simulink model "IEEE30_case"  (R2024b)
settings: Solver=FixedStepAuto  StartTime=0  StopTime=5  FixedStep=1e-7  RelTol=1e-3
values from neighbouring files (symbols this model uses):
  GFL_DFIG_7_C_bus = 0.08    [IEEE30_case_parameters.m]
  GFL_DFIG_7_D_mutual = 2.500000e+3    (= 2500)    [IEEE30_case_parameters.m]
  GFL_DFIG_7_f0 = 60    [IEEE30_case_parameters.m]
  GFL_DFIG_7_gPLLi = 3200    [IEEE30_case_parameters.m]
  GFL_DFIG_7_gPLLp = 650    [IEEE30_case_parameters.m]
  GFL_DFIG_7_H_WT = 0.4    [IEEE30_case_parameters.m]
  GFL_DFIG_7_Hg = 0.8    [IEEE30_case_parameters.m]
  GFL_DFIG_7_Igq_ref = 0    [IEEE30_case_parameters.m]
  GFL_DFIG_7_Ird_ref = 704.45696    [IEEE30_case_parameters.m]
  GFL_DFIG_7_KI_V = -300000    [IEEE30_case_parameters.m]
  GFL_DFIG_7_KP_V = -1000    [IEEE30_case_parameters.m]
  GFL_DFIG_7_Ksh = 1.254300e+4    (= 12543)    [IEEE30_case_parameters.m]
  GFL_DFIG_7_Lg = 0.000483    [IEEE30_case_parameters.m]
  GFL_DFIG_7_Lm_pu = 4    [IEEE30_case_parameters.m]
  GFL_DFIG_7_N = 100    [IEEE30_case_parameters.m]
  GFL_DFIG_7_p = 2    [IEEE30_case_parameters.m]
  GFL_DFIG_7_Pitch = 0    [IEEE30_case_parameters.m]
  GFL_DFIG_7_R = 44    [IEEE30_case_parameters.m]
  GFL_DFIG_7_Rg = 2.000000e-5    (= 2e-05)    [IEEE30_case_parameters.m]
  GFL_DFIG_7_rho = 1.225    [IEEE30_case_parameters.m]
  GFL_DFIG_7_rPLLi = 4500    [IEEE30_case_parameters.m]
  GFL_DFIG_7_rPLLp = 620    [IEEE30_case_parameters.m]
  GFL_DFIG_7_Rs_pu = 0.011    [IEEE30_case_parameters.m]
  GFL_DFIG_7_Sbase = 2.000000e+6    (= 2000000)    [IEEE30_case_parameters.m]
  GFL_DFIG_7_ugq_ref = 0    [IEEE30_case_parameters.m]
  GFL_DFIG_7_usd_ref = 0    [IEEE30_case_parameters.m]
  GFL_DFIG_7_Vbase = 690    [IEEE30_case_parameters.m]
  GFL_DFIG_7_Vdc_ref = 1200    [IEEE30_case_parameters.m]
  GFL_DFIG_7_wind = 12    [IEEE30_case_parameters.m]
  GFL_DFIG_7_wm_ref = 518.184209    [IEEE30_case_parameters.m]
  SG_D_13_D = 0.01056    [IEEE30_case_parameters.m]
  SG_D_13_EnableSaturation = 0    [IEEE30_case_parameters.m]
  SG_D_13_f0 = 60    [IEEE30_case_parameters.m]
  SG_D_13_H = 7.5    [IEEE30_case_parameters.m]
  SG_D_13_K_A = 20    [IEEE30_case_parameters.m]
  SG_D_13_K_E = 1.000000e+1    (= 10)    [IEEE30_case_parameters.m]
  SG_D_13_K_F = 2.363    [IEEE30_case_parameters.m]
  SG_D_13_K_s = 0.5    [IEEE30_case_parameters.m]
  SG_D_13_R_a = 0.001088    [IEEE30_case_parameters.m]
  SG_D_13_S_A = 1    [IEEE30_case_parameters.m]
  SG_D_13_S_B = 0.103    [IEEE30_case_parameters.m]
  SG_D_13_S_N = 10.659857    [IEEE30_case_parameters.m]
  SG_D_13_SpeedPara = 200    [IEEE30_case_parameters.m]
  SG_D_13_T_0 = 0.370163    [IEEE30_case_parameters.m]
  SG_D_13_T_1 = 0.3    [IEEE30_case_parameters.m]
  SG_D_13_T_2 = 0.05    [IEEE30_case_parameters.m]
  SG_D_13_T_3 = 0.02    [IEEE30_case_parameters.m]
  SG_D_13_T_4 = 0.005    [IEEE30_case_parameters.m]
  SG_D_13_T_A = 0.02    [IEEE30_case_parameters.m]
  SG_D_13_T_dd = 8.000000e+0    (= 8)    [IEEE30_case_parameters.m]
  SG_D_13_T_ddd = 0.04    [IEEE30_case_parameters.m]
  SG_D_13_T_E = 0.314    [IEEE30_case_parameters.m]
  SG_D_13_T_F = 0.35    [IEEE30_case_parameters.m]
  SG_D_13_T_qd = 0.8    [IEEE30_case_parameters.m]
  SG_D_13_T_qdd = 0.02    [IEEE30_case_parameters.m]
  SG_D_13_T_speed = 0.1    [IEEE30_case_parameters.m]
  SG_D_13_T_w = 0.5    [IEEE30_case_parameters.m]
  SG_D_13_V_ref = 1.696619    [IEEE30_case_parameters.m]
  SG_D_13_w_ref = 376.991118    [IEEE30_case_parameters.m]
  SG_D_13_x_d = 1.9    [IEEE30_case_parameters.m]
  SG_D_13_x_dd = 0.302    [IEEE30_case_parameters.m]
  SG_D_13_x_ddd = 0.204    [IEEE30_case_parameters.m]
  SG_D_13_x_l = 0.05    [IEEE30_case_parameters.m]
  SG_D_13_x_q = 1.3    [IEEE30_case_parameters.m]
  SG_D_13_x_qd = 0.5    [IEEE30_case_parameters.m]
  SG_D_13_x_qdd = 0.3    [IEEE30_case_parameters.m]
  SG_D_1_D = 0.01056    [IEEE30_case_parameters.m]
  SG_D_1_EnableSaturation = 0    [IEEE30_case_parameters.m]
  SG_D_1_f0 = 60    [IEEE30_case_parameters.m]
  SG_D_1_H = 7.5    [IEEE30_case_parameters.m]
  SG_D_1_K_A = 20    [IEEE30_case_parameters.m]
  SG_D_1_K_E = 1.000000e+1    (= 10)    [IEEE30_case_parameters.m]
  SG_D_1_K_F = 2.363    [IEEE30_case_parameters.m]
  SG_D_1_K_s = 0.5    [IEEE30_case_parameters.m]
  SG_D_1_R_a = 0.001088    [IEEE30_case_parameters.m]
  SG_D_1_S_A = 1    [IEEE30_case_parameters.m]
  SG_D_1_S_B = 0.103    [IEEE30_case_parameters.m]
  SG_D_1_S_N = 10.659857    [IEEE30_case_parameters.m]
  SG_D_1_SpeedPara = 200    [IEEE30_case_parameters.m]
  SG_D_1_T_0 = 0.259812    [IEEE30_case_parameters.m]
  SG_D_1_T_1 = 0.3    [IEEE30_case_parameters.m]
  SG_D_1_T_2 = 0.05    [IEEE30_case_parameters.m]
  SG_D_1_T_3 = 0.02    [IEEE30_case_parameters.m]
  SG_D_1_T_4 = 0.005    [IEEE30_case_parameters.m]
  SG_D_1_T_A = 0.02    [IEEE30_case_parameters.m]
  SG_D_1_T_dd = 8.000000e+0    (= 8)    [IEEE30_case_parameters.m]
  SG_D_1_T_ddd = 0.04    [IEEE30_case_parameters.m]
  SG_D_1_T_E = 0.314    [IEEE30_case_parameters.m]
  SG_D_1_T_F = 0.35    [IEEE30_case_parameters.m]
  SG_D_1_T_qd = 0.8    [IEEE30_case_parameters.m]
  SG_D_1_T_qdd = 0.02    [IEEE30_case_parameters.m]
  SG_D_1_T_speed = 0.1    [IEEE30_case_parameters.m]
  SG_D_1_T_w = 0.5    [IEEE30_case_parameters.m]
  SG_D_1_V_ref = 1.544107    [IEEE30_case_parameters.m]
  SG_D_1_w_ref = 376.991118    [IEEE30_case_parameters.m]
  SG_D_1_x_d = 1.9    [IEEE30_case_parameters.m]
  SG_D_1_x_dd = 0.302    [IEEE30_case_parameters.m]
  SG_D_1_x_ddd = 0.204    [IEEE30_case_parameters.m]
  SG_D_1_x_l = 0.05    [IEEE30_case_parameters.m]
  SG_D_1_x_q = 1.3    [IEEE30_case_parameters.m]
  SG_D_1_x_qd = 0.5    [IEEE30_case_parameters.m]
  SG_D_1_x_qdd = 0.3    [IEEE30_case_parameters.m]
  SG_D_22_D = 0.01056    [IEEE30_case_parameters.m]
  SG_D_22_EnableSaturation = 0    [IEEE30_case_parameters.m]
  SG_D_22_f0 = 60    [IEEE30_case_parameters.m]
  SG_D_22_H = 7.5    [IEEE30_case_parameters.m]
  SG_D_22_K_A = 20    [IEEE30_case_parameters.m]
  SG_D_22_K_E = 1.000000e+1    (= 10)    [IEEE30_case_parameters.m]
  SG_D_22_K_F = 2.363    [IEEE30_case_parameters.m]
  SG_D_22_K_s = 0.5    [IEEE30_case_parameters.m]
  SG_D_22_R_a = 0.001088    [IEEE30_case_parameters.m]
  SG_D_22_S_A = 1    [IEEE30_case_parameters.m]
  SG_D_22_S_B = 0.103    [IEEE30_case_parameters.m]
  SG_D_22_S_N = 10.659857    [IEEE30_case_parameters.m]
  SG_D_22_SpeedPara = 200    [IEEE30_case_parameters.m]
  SG_D_22_T_0 = 0.216121    [IEEE30_case_parameters.m]
  SG_D_22_T_1 = 0.3    [IEEE30_case_parameters.m]
  SG_D_22_T_2 = 0.05    [IEEE30_case_parameters.m]
  SG_D_22_T_3 = 0.02    [IEEE30_case_parameters.m]
  SG_D_22_T_4 = 0.005    [IEEE30_case_parameters.m]
  ... (+126 more)
(part 22 of 27)

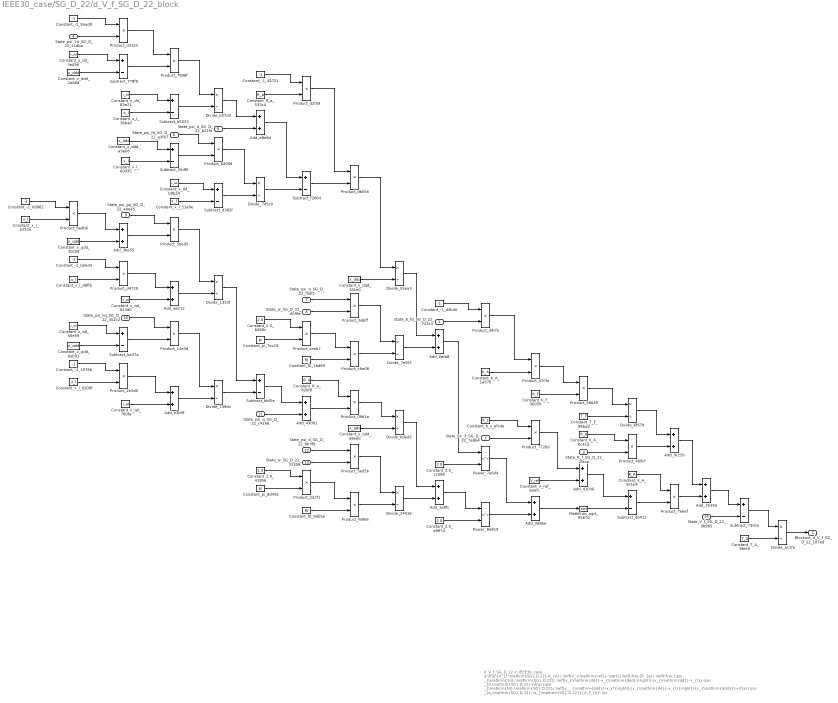
== system IEEE30_case/SG_D_22/d_V_f_SG_D_22_block ==
  note: d_V_f_SG_D_22 in IEEE30_case
      | $-\frac{V_{f,\mathrm{SG},D,22}-K_{A}\,\left(V_{\mathrm{ref}}-\sqrt{{\left(\frac{R_{a}\,\left(\frac{\psi _{\mathrm{1d},\mathrm{SG},D,22}\,\left(x_{\mathrm{dd}}-x_{\mathrm{ddd}}\right)}{x_{\mathrm{dd}}-x_{l}}-\psi _{d,\mathrm{SG},D,22}+\frac{\psi _{\mathrm{fd},\mathrm{SG},D,22}\,\left(x_{\mathrm{ddd}}-x_{l}\right)}{x_{\mathrm{dd}}-x_{l}}\right)}{x_{\mathrm{ddd}}}+\frac{\psi _{q,\mathrm{SG},D,22}\,w_{\mathrm{SG},D,22}}{2\,f_{0}\,\pi }\right)}^2+{\left(\frac{R_{a}\,\left(\psi _{q,\mathrm{SG},D,22}+\frac{\psi _{\mathrm{gq},\mathrm{SG},D,22}\,\left(x_{l}-x_{\mathrm{qdd}}\right)}{x_{l}-x_{\mathrm{qd}}}+\frac{\psi _{\mathrm{kq},\mathrm{SG},D,22}\,\left(x_{\mathrm{qd}}-x_{\mathrm{qdd}}\right)}{x_{l}-x_{\mathrm{qd}}}\right)}{x_{\mathrm{qdd}}}+\frac{\psi _{d,\mathrm{SG},D,22}\,w_{\mathrm{SG},D,22}}{2\,f_{0}\,\pi }\right)}^2}+K_{s}\,\mathrm{Px}_{3,\mathrm{SG},D,22}\right)-K_{A}\,R_{f,\mathrm{SG},D,22}+\frac{E_{\mathrm{fd},\mathrm{SG},D,22}\,K_{A}\,K_{F}}{T_{F}}}{T_{A}}$
      | Automatically generated on 2025-11-01 18:36:26 .
  State_E_fd_SG_D_22_743c3 : Inport
  State_R_f_SG_D_22_2faca : Inport  Port=2
  State_Px_3_SG_D_22_7a9b4 : Inport  Port=3
  State_psi_1d_SG_D_22_11dba : Inport  Port=4
  State_psi_d_SG_D_22_b21fa : Inport  Port=5
  State_psi_fd_SG_D_22_e3f07 : Inport  Port=6
  State_psi_q_SG_D_22_f5df1 : Inport  Port=7
  State_w_SG_D_22_d59fe : Inport  Port=8
  State_psi_gq_SG_D_22_abe45 : Inport  Port=9
  State_psi_kq_SG_D_22_352c2 : Inport  Port=10
  State_psi_q_SG_D_22_c4168 : Inport  Port=11
  State_psi_d_SG_D_22_8b3f8 : Inport  Port=12
  State_w_SG_D_22_31356 : Inport  Port=13
  State_V_f_SG_D_22_db965 : Inport  Port=14
  Add_0efa8 : Sum
  Add_1e8fc : Sum
  Add_3539d : Sum
  Add_3be55 : Sum
  Add_3d8ee : Sum
  Add_41036 : Sum
  Add_43081 : Sum
  Add_9cc50 : Sum
  Add_a6212 : Sum
  Add_e3b9f : Sum
  Add_e8e6d : Sum
  Constant_-1_0d962 : Constant  Value=-1
  Constant_-1_1978b : Constant  Value=-1
  Constant_-1_44751 : Constant  Value=-1
  Constant_-1_9aad8 : Constant  Value=-1
  Constant_-1_bb5d4 : Constant  Value=-1
  Constant_-1_d3b46 : Constant  Value=-1
  Constant_2.0_41856 : Constant  Value=2.0
  Constant_2.0_a9874 : Constant  Value=2.0
  Constant_2.0_b068c : Constant  Value=2.0
  Constant_2.0_cc098 : Constant  Value=2.0
  Constant_K_A_0c41a : Constant  Value=K_A
  Constant_K_A_1a676 : Constant  Value=K_A
  Constant_K_A_8c1b4 : Constant  Value=K_A
  Constant_K_F_36050 : Constant  Value=K_F
  Constant_K_s_afc4e : Constant  Value=K_s
  Constant_R_a_533c4 : Constant  Value=R_a
  Constant_R_a_82bf8 : Constant  Value=R_a
  Constant_T_A_9fe59 : Constant  Value=T_A
  Constant_T_F_98bad : Constant  Value=T_F
  Constant_V_ref_6e5fc : Constant  Value=V_ref
  Constant_f0_1bd69 : Constant  Value=f0
  Constant_f0_9db5e : Constant  Value=f0
  Constant_pi_7ac18 : Constant  Value=pi
  Constant_pi_8d43a : Constant  Value=pi
  Constant_x_dd_83e21 : Constant  Value=x_dd
  Constant_x_dd_b9b24 : Constant  Value=x_dd
  Constant_x_dd_fe496 : Constant  Value=x_dd
  Constant_x_ddd_191e0 : Constant  Value=x_ddd
  Constant_x_ddd_2a6b8 : Constant  Value=x_ddd
  Constant_x_ddd_a3e68 : Constant  Value=x_ddd
  Constant_x_l_38b4d : Constant  Value=x_l
  Constant_x_l_51a9e : Constant  Value=x_l
  Constant_x_l_60d35 : Constant  Value=x_l
  Constant_x_l_d208f : Constant  Value=x_l
  Constant_x_l_d6ffb : Constant  Value=x_l
  Constant_x_l_e152e : Constant  Value=x_l
  Constant_x_qd_56e59 : Constant  Value=x_qd
  Constant_x_qd_760fa : Constant  Value=x_qd
  Constant_x_qd_813d0 : Constant  Value=x_qd
  Constant_x_qdd_0eb91 : Constant  Value=x_qdd
  Constant_x_qdd_30cb9 : Constant  Value=x_qdd
  Constant_x_qdd_d8eeb : Constant  Value=x_qdd
  Divide_1353f : Product  Inputs=*/
  Divide_24016 : Product  Inputs=*/
  Divide_55ea3 : Product  Inputs=*/
  Divide_6f679 : Product  Inputs=*/
  Divide_749cb : Product  Inputs=*/
  Divide_7d5c0 : Product  Inputs=*/
  Divide_7e91f : Product  Inputs=*/
  Divide_ac1fa : Product  Inputs=*/
  Divide_b57d3 : Product  Inputs=*/
  Divide_bded9 : Product  Inputs=*/
  MathFunc_sqrt_95670 : Sqrt
  Power_7a6d4 : Math  Operator=pow
  Power_8e819 : Math  Operator=pow
  Product_0961a : Product
  Product_14e3d : Product
  Product_2d2f1 : Product
  Product_2e2d0 : Product
  Product_469cf : Product
  Product_47f3a : Product
  Product_56649 : Product
  Product_5ed5b : Product
  Product_5eed5 : Product
  Product_6409d : Product
  Product_7726d : Product
  Product_7848f : Product
  Product_7e6ef : Product
  Product_8adb6 : Product
  Product_9dbff : Product
  Product_c6e08 : Product
  Product_ceab7 : Product
  Product_d2f59 : Product
  Product_d31e3 : Product
  Product_d4729 : Product
  Product_d4cfa : Product
  Product_db056 : Product
  Product_f69e6 : Product
  Subtract_35df0 : Sum  Inputs=+-
  Subtract_730ce : Sum  Inputs=+-
  Subtract_778f9 : Sum  Inputs=+-
  Subtract_b5033 : Sum  Inputs=+-
  Subtract_ba37a : Sum  Inputs=+-
  Subtract_bbf2a : Sum  Inputs=+-
  Subtract_d0412 : Sum  Inputs=+-
  Subtract_d382f : Sum  Inputs=+-
  Subtract_f2864 : Sum  Inputs=+-
  Blockout_d_V_f_SG_D_22_187ed : Outport
  wires:
  Constant_-1_0d962/1 -> Product_8adb6/1
  Product_8adb6/1 -> Add_3be55/1
  Constant_x_l_e152e/1 -> Product_8adb6/2
  Product_d31e3/1 -> Product_7848f/1
  Constant_-1_9aad8/1 -> Product_d31e3/1
  Subtract_778f9/1 -> Product_7848f/2
  Constant_x_dd_fe496/1 -> Subtract_778f9/1
  Product_6409d/1 -> Divide_7d5c0/1
  State_psi_1d_SG_D_22_11dba/1 -> Product_d31e3/2
  Constant_x_qdd_30cb9/1 -> Add_3be55/2
  State_psi_q_SG_D_22_f5df1/1 -> Product_9dbff/1
  Constant_x_ddd_2a6b8/1 -> Subtract_778f9/2
  Product_d4729/1 -> Add_a6212/1
  Constant_-1_bb5d4/1 -> Product_d4729/1
  Product_ceab7/1 -> Product_c6e08/1
  Constant_x_l_d6ffb/1 -> Product_d4729/2
  Constant_2.0_b068c/1 -> Product_ceab7/1
  Subtract_ba37a/1 -> Product_14e3d/2
  Constant_x_qd_56e59/1 -> Subtract_ba37a/1
  Subtract_bbf2a/1 -> Add_43081/1
  Constant_x_qdd_0eb91/1 -> Subtract_ba37a/2
  Constant_-1_44751/1 -> Product_d2f59/1
  Product_2e2d0/1 -> Add_e3b9f/1
  Constant_-1_1978b/1 -> Product_2e2d0/1
  Constant_x_dd_b9b24/1 -> Subtract_d382f/1
  Constant_x_l_d208f/1 -> Product_2e2d0/2
  Constant_2.0_41856/1 -> Product_2d2f1/1
  Subtract_b5033/1 -> Divide_b57d3/2
  Constant_x_dd_83e21/1 -> Subtract_b5033/1
  Constant_pi_8d43a/1 -> Product_2d2f1/2
  Constant_x_l_38b4d/1 -> Subtract_b5033/2
  Constant_x_qd_760fa/1 -> Add_e3b9f/2
  Constant_x_ddd_a3e68/1 -> Subtract_35df0/1
  Subtract_f2864/1 -> Product_db056/2
  Constant_x_l_60d35/1 -> Subtract_35df0/2
  Product_5eed5/1 -> Divide_1353f/1
  State_psi_gq_SG_D_22_abe45/1 -> Product_5eed5/1
  Add_3be55/1 -> Product_5eed5/2
  Constant_x_qd_813d0/1 -> Add_a6212/2
  Product_14e3d/1 -> Divide_749cb/1
  State_psi_kq_SG_D_22_352c2/1 -> Product_14e3d/1
  Product_7848f/1 -> Divide_b57d3/1
  State_psi_fd_SG_D_22_e3f07/1 -> Product_6409d/1
  State_psi_q_SG_D_22_c4168/1 -> Add_43081/2
  Subtract_35df0/1 -> Product_6409d/2
  Constant_x_l_51a9e/1 -> Subtract_d382f/2
  Constant_f0_1bd69/1 -> Product_c6e08/2
  Add_a6212/1 -> Divide_1353f/2
  Product_d2f59/1 -> Product_db056/1
  Add_e3b9f/1 -> Divide_749cb/2
  Divide_b57d3/1 -> Add_e8e6d/1
  State_psi_d_SG_D_22_b21fa/1 -> Add_e8e6d/2
  Constant_R_a_533c4/1 -> Product_d2f59/2
  Subtract_d382f/1 -> Divide_7d5c0/2
  Divide_1353f/1 -> Subtract_bbf2a/1
  Divide_749cb/1 -> Subtract_bbf2a/2
  Add_e8e6d/1 -> Subtract_f2864/1
  Divide_7d5c0/1 -> Subtract_f2864/2
  Constant_pi_7ac18/1 -> Product_ceab7/2
  State_w_SG_D_22_d59fe/1 -> Product_9dbff/2
  Constant_R_a_82bf8/1 -> Product_0961a/1
  Add_43081/1 -> Product_0961a/2
  State_psi_d_SG_D_22_8b3f8/1 -> Product_5ed5b/1
  State_w_SG_D_22_31356/1 -> Product_5ed5b/2
  Product_2d2f1/1 -> Product_f69e6/1
  Constant_f0_9db5e/1 -> Product_f69e6/2
  Product_db056/1 -> Divide_55ea3/1
  Constant_x_ddd_191e0/1 -> Divide_55ea3/2
  Product_9dbff/1 -> Divide_7e91f/1
  Product_c6e08/1 -> Divide_7e91f/2
  Product_0961a/1 -> Divide_bded9/1
  Constant_x_qdd_d8eeb/1 -> Divide_bded9/2
  Product_5ed5b/1 -> Divide_24016/1
  Product_f69e6/1 -> Divide_24016/2
  Constant_K_A_1a676/1 -> Product_47f3a/2
  Divide_55ea3/1 -> Add_0efa8/1
  Divide_7e91f/1 -> Add_0efa8/2
  Divide_bded9/1 -> Add_1e8fc/1
  Divide_24016/1 -> Add_1e8fc/2
  Constant_-1_d3b46/1 -> Product_d4cfa/1
  State_E_fd_SG_D_22_743c3/1 -> Product_d4cfa/2
  Add_0efa8/1 -> Power_7a6d4/1
  Constant_2.0_cc098/1 -> Power_7a6d4/2
  Add_1e8fc/1 -> Power_8e819/1
  Constant_2.0_a9874/1 -> Power_8e819/2
  Product_d4cfa/1 -> Product_47f3a/1
  Constant_K_s_afc4e/1 -> Product_7726d/1
  State_Px_3_SG_D_22_7a9b4/1 -> Product_7726d/2
  Power_7a6d4/1 -> Add_3d8ee/1
  Power_8e819/1 -> Add_3d8ee/2
  Product_47f3a/1 -> Product_56649/1
  Add_3d8ee/1 -> MathFunc_sqrt_95670/1
  Constant_K_F_36050/1 -> Product_56649/2
  Product_7726d/1 -> Add_41036/1
  Constant_V_ref_6e5fc/1 -> Add_41036/2
  Product_56649/1 -> Divide_6f679/1
  Constant_T_F_98bad/1 -> Divide_6f679/2
  Constant_K_A_0c41a/1 -> Product_469cf/1
  State_R_f_SG_D_22_2faca/1 -> Product_469cf/2
  Add_41036/1 -> Subtract_d0412/1
  MathFunc_sqrt_95670/1 -> Subtract_d0412/2
  Divide_6f679/1 -> Add_9cc50/1
  Product_469cf/1 -> Add_9cc50/2
  Constant_K_A_8c1b4/1 -> Product_7e6ef/1
  Subtract_d0412/1 -> Product_7e6ef/2
  Add_9cc50/1 -> Add_3539d/1
  Product_7e6ef/1 -> Add_3539d/2
  Add_3539d/1 -> Subtract_730ce/1
  State_V_f_SG_D_22_db965/1 -> Subtract_730ce/2
  Subtract_730ce/1 -> Divide_ac1fa/1
  Constant_T_A_9fe59/1 -> Divide_ac1fa/2
  Divide_ac1fa/1 -> Blockout_d_V_f_SG_D_22_187ed/1

== system IEEE30_case/SG_D_22/d_psi_1d_SG_D_22_block ==
  note: d_psi_1d_SG_D_22 in IEEE30_case
      | $-\frac{\psi _{\mathrm{1d},\mathrm{SG},D,22}-\psi _{\mathrm{fd},\mathrm{SG},D,22}+\frac{\left(x_{\mathrm{dd}}-x_{l}\right)\,\left(\frac{\psi _{\mathrm{1d},\mathrm{SG},D,22}\,\left(x_{\mathrm{dd}}-x_{\mathrm{ddd}}\right)}{x_{\mathrm{dd}}-x_{l}}-\psi _{d,\mathrm{SG},D,22}+\frac{\psi _{\mathrm{fd},\mathrm{SG},D,22}\,\left(x_{\mathrm{ddd}}-x_{l}\right)}{x_{\mathrm{dd}}-x_{l}}\right)}{x_{\mathrm{ddd}}}}{T_{\mathrm{ddd}}}$
      | Automatically generated on 2025-11-01 18:36:01 .
  State_psi_1d_SG_D_22_172da : Inport
  State_psi_fd_SG_D_22_c2d5a : Inport  Port=2
  State_psi_1d_SG_D_22_e0ab6 : Inport  Port=3
  State_psi_d_SG_D_22_a4972 : Inport  Port=4
  State_psi_fd_SG_D_22_3322a : Inport  Port=5
  Add_5a731 : Sum
  Add_823bb : Sum
  Add_8bdee : Sum
  Constant_-1_43b70 : Constant  Value=-1
  Constant_-1_e3690 : Constant  Value=-1
  Constant_T_ddd_16786 : Constant  Value=T_ddd
  Constant_x_dd_2a533 : Constant  Value=x_dd
  Constant_x_dd_3a236 : Constant  Value=x_dd
  Constant_x_dd_89937 : Constant  Value=x_dd
  Constant_x_dd_d0c64 : Constant  Value=x_dd
  Constant_x_ddd_40c6f : Constant  Value=x_ddd
  Constant_x_ddd_7eefb : Constant  Value=x_ddd
  Constant_x_ddd_b7266 : Constant  Value=x_ddd
  Constant_x_l_19e50 : Constant  Value=x_l
  Constant_x_l_5eccd : Constant  Value=x_l
  Constant_x_l_88938 : Constant  Value=x_l
  Constant_x_l_d4803 : Constant  Value=x_l
  Divide_10e07 : Product  Inputs=*/
  Divide_5218a : Product  Inputs=*/
  Divide_a8712 : Product  Inputs=*/
  Divide_da239 : Product  Inputs=*/
  Product_011ec : Product
  Product_57d84 : Product
  Product_6887b : Product
  Product_99b88 : Product
  Product_9d3cd : Product
  Subtract_1db70 : Sum  Inputs=+-
  Subtract_59386 : Sum  Inputs=+-
  Subtract_5a27d : Sum  Inputs=+-
  Subtract_b5060 : Sum  Inputs=+-
  Subtract_b7795 : Sum  Inputs=+-
  Subtract_e43cc : Sum  Inputs=+-
  Blockout_d_psi_1d_SG_D_22_39dbc : Outport
  wires:
  Constant_-1_e3690/1 -> Product_9d3cd/1
  State_psi_1d_SG_D_22_e0ab6/1 -> Product_9d3cd/2
  Constant_x_l_88938/1 -> Subtract_59386/2
  Subtract_b5060/1 -> Product_6887b/2
  Constant_x_dd_2a533/1 -> Subtract_1db70/1
  Product_9d3cd/1 -> Product_99b88/1
  Divide_5218a/1 -> Subtract_5a27d/2
  Constant_x_ddd_40c6f/1 -> Subtract_1db70/2
  Subtract_1db70/1 -> Product_99b88/2
  State_psi_d_SG_D_22_a4972/1 -> Add_8bdee/2
  Subtract_b7795/1 -> Divide_da239/2
  Constant_x_dd_89937/1 -> Subtract_b7795/1
  Constant_x_l_d4803/1 -> Subtract_b7795/2
  Constant_x_ddd_b7266/1 -> Subtract_b5060/1
  Add_5a731/1 -> Divide_a8712/1
  Constant_x_l_5eccd/1 -> Subtract_b5060/2
  Product_99b88/1 -> Divide_da239/1
  State_psi_fd_SG_D_22_3322a/1 -> Product_6887b/1
  Constant_x_dd_3a236/1 -> Subtract_e43cc/1
  Constant_x_l_19e50/1 -> Subtract_e43cc/2
  Divide_da239/1 -> Add_8bdee/1
  Product_6887b/1 -> Divide_5218a/1
  Subtract_e43cc/1 -> Divide_5218a/2
  Constant_x_dd_d0c64/1 -> Subtract_59386/1
  Add_8bdee/1 -> Subtract_5a27d/1
  Constant_-1_43b70/1 -> Product_011ec/1
  Add_823bb/1 -> Add_5a731/1
  State_psi_1d_SG_D_22_172da/1 -> Product_011ec/2
  Subtract_59386/1 -> Product_57d84/1
  Divide_10e07/1 -> Add_5a731/2
  Subtract_5a27d/1 -> Product_57d84/2
  Product_011ec/1 -> Add_823bb/1
  State_psi_fd_SG_D_22_c2d5a/1 -> Add_823bb/2
  Product_57d84/1 -> Divide_10e07/1
  Constant_x_ddd_7eefb/1 -> Divide_10e07/2
  Divide_a8712/1 -> Blockout_d_psi_1d_SG_D_22_39dbc/1
  Constant_T_ddd_16786/1 -> Divide_a8712/2

== system IEEE30_case/SG_D_22/d_psi_d_SG_D_22_block ==
  note: d_psi_d_SG_D_22 in IEEE30_case
      | $2\,\pi \,f_{0}\,\left(v_{d,\mathrm{SG},D,22}\,\sin\left(\theta _{\mathrm{SG},D,22}\right)-v_{q,\mathrm{SG},D,22}\,\cos\left(\theta _{\mathrm{SG},D,22}\right)+\frac{R_{a}\,\left(\frac{\psi _{\mathrm{1d},\mathrm{SG},D,22}\,\left(x_{\mathrm{dd}}-x_{\mathrm{ddd}}\right)}{x_{\mathrm{dd}}-x_{l}}-\psi _{d,\mathrm{SG},D,22}+\frac{\psi _{\mathrm{fd},\mathrm{SG},D,22}\,\left(x_{\mathrm{ddd}}-x_{l}\right)}{x_{\mathrm{dd}}-x_{l}}\right)}{x_{\mathrm{ddd}}}+\frac{\psi _{q,\mathrm{SG},D,22}\,w_{\mathrm{SG},D,22}}{2\,f_{0}\,\pi }\right)$
      | Automatically generated on 2025-11-01 18:35:50 .
  State_psi_1d_SG_D_22_f0d35 : Inport
  State_psi_d_SG_D_22_c5170 : Inport  Port=2
  State_psi_fd_SG_D_22_05db2 : Inport  Port=3
  Input_v_d_SG_D_22_73bdd : Inport  Port=4
  State_theta_SG_D_22_96219 : Inport  Port=5
  Input_v_q_SG_D_22_3bdb8 : Inport  Port=6
  State_theta_SG_D_22_18f7d : Inport  Port=7
  State_psi_q_SG_D_22_e1063 : Inport  Port=8
  State_w_SG_D_22_ad5b4 : Inport  Port=9
  Add_9f87f : Sum
  Add_ed00b : Sum
  Constant_-1_4b6c9 : Constant  Value=-1
  Constant_-2.0_fe80e : Constant  Value=-2.0
  Constant_2.0_3d0f3 : Constant  Value=2.0
  Constant_R_a_1a13e : Constant  Value=R_a
  Constant_f0_968cd : Constant  Value=f0
  Constant_f0_e2609 : Constant  Value=f0
  Constant_pi_aa993 : Constant  Value=pi
  Constant_pi_f766b : Constant  Value=pi
  Constant_x_dd_37716 : Constant  Value=x_dd
  Constant_x_dd_9988e : Constant  Value=x_dd
  Constant_x_dd_ac2eb : Constant  Value=x_dd
  Constant_x_ddd_1a8f3 : Constant  Value=x_ddd
  Constant_x_ddd_2ce2e : Constant  Value=x_ddd
  Constant_x_ddd_ed9b0 : Constant  Value=x_ddd
  Constant_x_l_11583 : Constant  Value=x_l
  Constant_x_l_647b1 : Constant  Value=x_l
  Constant_x_l_e8c79 : Constant  Value=x_l
  Divide_06016 : Product  Inputs=*/
  Divide_571ed : Product  Inputs=*/
  Divide_b6e6b : Product  Inputs=*/
  Divide_f6f7e : Product  Inputs=*/
  MathFunc_cos_c55f9 : Trigonometry  Operator=cos
  MathFunc_sin_e4025 : Trigonometry
  Product_0567a : Product
  Product_0aaf0 : Product
  Product_0e150 : Product
  Product_18bce : Product
  Product_1f800 : Product
  Product_30e33 : Product
  Product_4a35a : Product
  Product_{56643,75402,80590,84044} (4 alike) : Product
  Product_73c43 : Product
  Subtract_40475 : Sum  Inputs=+-
  Subtract_424d8 : Sum  Inputs=+-
  Subtract_6dd7a : Sum  Inputs=+-
  Subtract_8ad17 : Sum  Inputs=+-
  Subtract_b2395 : Sum  Inputs=+-
  Subtract_d7e71 : Sum  Inputs=+-
  Subtract_d9587 : Sum  Inputs=+-
  Blockout_d_psi_d_SG_D_22_244d3 : Outport
  wires:
  Constant_-1_4b6c9/1 -> Product_80590/1
  Product_80590/1 -> Product_30e33/1
  Constant_x_dd_37716/1 -> Subtract_d9587/1
  Subtract_d9587/1 -> Product_30e33/2
  State_psi_1d_SG_D_22_f0d35/1 -> Product_80590/2
  Constant_f0_968cd/1 -> Product_56643/2
  Subtract_d7e71/1 -> Divide_571ed/2
  Constant_x_dd_9988e/1 -> Subtract_d7e71/1
  Subtract_b2395/1 -> Product_75402/2
  Constant_x_ddd_ed9b0/1 -> Subtract_d9587/2
  Constant_x_l_11583/1 -> Subtract_d7e71/2
  Product_56643/1 -> Product_75402/1
  Subtract_8ad17/1 -> Product_4a35a/2
  Constant_x_ddd_1a8f3/1 -> Subtract_8ad17/1
  Constant_x_l_647b1/1 -> Subtract_8ad17/2
  Product_30e33/1 -> Divide_571ed/1
  Product_4a35a/1 -> Divide_b6e6b/1
  State_psi_fd_SG_D_22_05db2/1 -> Product_4a35a/1
  Subtract_424d8/1 -> Divide_b6e6b/2
  Constant_x_dd_ac2eb/1 -> Subtract_424d8/1
  MathFunc_cos_c55f9/1 -> Product_73c43/2
  State_theta_SG_D_22_18f7d/1 -> MathFunc_cos_c55f9/1
  Constant_x_l_e8c79/1 -> Subtract_424d8/2
  Divide_571ed/1 -> Add_9f87f/1
  Product_18bce/1 -> Product_56643/1
  State_psi_d_SG_D_22_c5170/1 -> Add_9f87f/2
  Add_9f87f/1 -> Subtract_6dd7a/1
  State_w_SG_D_22_ad5b4/1 -> Product_0aaf0/2
  Divide_b6e6b/1 -> Subtract_6dd7a/2
  Product_1f800/1 -> Divide_06016/1
  Constant_R_a_1a13e/1 -> Product_1f800/1
  Subtract_6dd7a/1 -> Product_1f800/2
  Constant_f0_e2609/1 -> Product_0567a/2
  State_theta_SG_D_22_96219/1 -> MathFunc_sin_e4025/1
  Constant_x_ddd_2ce2e/1 -> Divide_06016/2
  Input_v_d_SG_D_22_73bdd/1 -> Product_0e150/1
  Constant_pi_f766b/1 -> Product_84044/2
  MathFunc_sin_e4025/1 -> Product_0e150/2
  Product_84044/1 -> Product_0567a/1
  Constant_2.0_3d0f3/1 -> Product_84044/1
  Divide_06016/1 -> Subtract_40475/1
  Product_0e150/1 -> Subtract_40475/2
  Product_73c43/1 -> Add_ed00b/2
  Input_v_q_SG_D_22_3bdb8/1 -> Product_73c43/1
  State_psi_q_SG_D_22_e1063/1 -> Product_0aaf0/1
  Constant_-2.0_fe80e/1 -> Product_18bce/1
  Constant_pi_aa993/1 -> Product_18bce/2
  Subtract_40475/1 -> Add_ed00b/1
  Product_0aaf0/1 -> Divide_f6f7e/1
  Product_0567a/1 -> Divide_f6f7e/2
  Add_ed00b/1 -> Subtract_b2395/1
  Divide_f6f7e/1 -> Subtract_b2395/2
  Product_75402/1 -> Blockout_d_psi_d_SG_D_22_244d3/1

== system IEEE30_case/SG_D_22/d_psi_fd_SG_D_22_block ==
  note: d_psi_fd_SG_D_22 in IEEE30_case
      | $-\frac{\psi _{\mathrm{fd},\mathrm{SG},D,22}-E_{\mathrm{fd},\mathrm{SG},D,22}+\left(x_{d}-x_{\mathrm{dd}}\right)\,\left(\frac{\frac{\psi _{\mathrm{1d},\mathrm{SG},D,22}\,\left(x_{\mathrm{dd}}-x_{\mathrm{ddd}}\right)}{x_{\mathrm{dd}}-x_{l}}-\psi _{d,\mathrm{SG},D,22}+\frac{\psi _{\mathrm{fd},\mathrm{SG},D,22}\,\left(x_{\mathrm{ddd}}-x_{l}\right)}{x_{\mathrm{dd}}-x_{l}}}{x_{\mathrm{ddd}}}-\frac{\left(x_{\mathrm{dd}}-x_{\mathrm{ddd}}\right)\,\left(\psi _{\mathrm{1d},\mathrm{SG},D,22}-\psi _{\mathrm{fd},\mathrm{SG},D,22}+\frac{\left(x_{\mathrm{dd}}-x_{l}\right)\,\left(\frac{\psi _{\mathrm{1d},\mathrm{SG},D,22}\,\left(x_{\mathrm{dd}}-x_{\mathrm{ddd}}\right)}{x_{\mathrm{dd}}-x_{l}}-\psi _{d,\mathrm{SG},D,22}+\frac{\psi _{\mathrm{fd},\mathrm{SG},D,22}\,\left(x_{\mathrm{ddd}}-x_{l}\right)}{x_{\mathrm{dd}}-x_{l}}\right)}{x_{\mathrm{ddd}}}\right)}{{\left(x_{\mathrm{dd}}-x_{l}\right)}^2}\right)}{T_{\mathrm{dd}}}$
      | Automatically generated on 2025-11-01 18:35:58 .
  State_E_fd_SG_D_22_516e7 : Inport
  State_psi_fd_SG_D_22_5b8ee : Inport  Port=2
  State_psi_1d_SG_D_22_be8ba : Inport  Port=3
  State_psi_fd_SG_D_22_f44ac : Inport  Port=4
  State_psi_1d_SG_D_22_63a8d : Inport  Port=5
  State_psi_d_SG_D_22_1ab68 : Inport  Port=6
  State_psi_fd_SG_D_22_b3331 : Inport  Port=7
  State_psi_1d_SG_D_22_ea7d2 : Inport  Port=8
  State_psi_d_SG_D_22_f7c75 : Inport  Port=9
  State_psi_fd_SG_D_22_ee685 : Inport  Port=10
  Add_26b3d : Sum
  Add_db1cd : Sum
  Constant_-1_236d3 : Constant  Value=-1
  Constant_-1_84c87 : Constant  Value=-1
  Constant_-1_be10d : Constant  Value=-1
  Constant_2.0_3cf32 : Constant  Value=2.0
  Constant_T_dd_0394b : Constant  Value=T_dd
  Constant_x_d_d871a : Constant  Value=x_d
  Constant_x_dd_234ce : Constant  Value=x_dd
  Constant_x_dd_31f3c : Constant  Value=x_dd
  Constant_x_dd_429ce : Constant  Value=x_dd
  Constant_x_dd_60a36 : Constant  Value=x_dd
  Constant_x_dd_7d927 : Constant  Value=x_dd
  Constant_x_dd_b910b : Constant  Value=x_dd
  Constant_x_dd_d9ba6 : Constant  Value=x_dd
  Constant_x_dd_e67fe : Constant  Value=x_dd
  Constant_x_dd_effc2 : Constant  Value=x_dd
  Constant_x_dd_f4ac1 : Constant  Value=x_dd
  Constant_x_ddd_1b0fe : Constant  Value=x_ddd
  Constant_x_ddd_1deae : Constant  Value=x_ddd
  Constant_x_ddd_21800 : Constant  Value=x_ddd
  Constant_x_ddd_282e7 : Constant  Value=x_ddd
  Constant_x_ddd_45fea : Constant  Value=x_ddd
  Constant_x_ddd_ce638 : Constant  Value=x_ddd
  Constant_x_ddd_e54ea : Constant  Value=x_ddd
  Constant_x_l_025b1 : Constant  Value=x_l
  Constant_x_l_0af95 : Constant  Value=x_l
  Constant_x_l_441e6 : Constant  Value=x_l
  Constant_x_l_4809b : Constant  Value=x_l
  Constant_x_l_4e88b : Constant  Value=x_l
  Constant_x_l_8603d : Constant  Value=x_l
  Constant_x_l_9a4a1 : Constant  Value=x_l
  Constant_x_l_d68d3 : Constant  Value=x_l
  Divide_05403 : Product  Inputs=*/
  Divide_2963f : Product  Inputs=*/
  Divide_58225 : Product  Inputs=*/
  Divide_a0f43 : Product  Inputs=*/
  Divide_b3bbc : Product  Inputs=*/
  Divide_e4323 : Product  Inputs=*/
  Divide_eeebf : Product  Inputs=*/
  Divide_f671b : Product  Inputs=*/
  Power_fbb4c : Math  Operator=pow
  Product_0db9f : Product
  Product_1b057 : Product
  Product_72ee2 : Product
  Product_8dcb9 : Product
  Product_95cd6 : Product
  Product_9c35a : Product
  Product_9e2dc : Product
  Product_acfc4 : Product
  Product_b2552 : Product
  Product_f9d7f : Product
  Subtract_04006 : Sum  Inputs=+-
  Subtract_0684c : Sum  Inputs=+-
  Subtract_12a24 : Sum  Inputs=+-
  Subtract_1a20e : Sum  Inputs=+-
  Subtract_298af : Sum  Inputs=+-
  Subtract_362e6 : Sum  Inputs=+-
  Subtract_3cffd : Sum  Inputs=+-
  Subtract_47005 : Sum  Inputs=+-
  Subtract_4e4d5 : Sum  Inputs=+-
  Subtract_5b279 : Sum  Inputs=+-
  Subtract_5f8ae : Sum  Inputs=+-
  Subtract_6847d : Sum  Inputs=+-
  Subtract_6b974 : Sum  Inputs=+-
  Subtract_6c244 : Sum  Inputs=+-
  Subtract_8d9fd : Sum  Inputs=+-
  Subtract_9e44c : Sum  Inputs=+-
  Subtract_af608 : Sum  Inputs=+-
  Subtract_b0387 : Sum  Inputs=+-
  Subtract_f2eb4 : Sum  Inputs=+-
  Blockout_d_psi_fd_SG_D_22_1ac55 : Outport
  wires:
  Constant_-1_236d3/1 -> Product_9e2dc/1
  Product_9e2dc/1 -> Product_b2552/1
  Constant_x_dd_234ce/1 -> Subtract_298af/1
  Subtract_298af/1 -> Product_b2552/2
  State_psi_1d_SG_D_22_63a8d/1 -> Product_9e2dc/2
  Constant_x_dd_429ce/1 -> Subtract_6b974/1
  Constant_x_ddd_ce638/1 -> Subtract_298af/2
  Subtract_3cffd/1 -> Divide_b3bbc/2
  Constant_x_dd_7d927/1 -> Subtract_3cffd/1
  Constant_x_l_0af95/1 -> Subtract_3cffd/2
  Constant_x_ddd_282e7/1 -> Subtract_b0387/1
  Subtract_47005/1 -> Divide_58225/2
  Constant_x_l_441e6/1 -> Subtract_b0387/2
  Product_b2552/1 -> Divide_b3bbc/1
  State_E_fd_SG_D_22_516e7/1 -> Subtract_5b279/1
  State_psi_fd_SG_D_22_b3331/1 -> Product_acfc4/1
  Subtract_b0387/1 -> Product_acfc4/2
  Constant_x_dd_60a36/1 -> Subtract_47005/1
  Product_acfc4/1 -> Divide_58225/1
  Constant_x_l_9a4a1/1 -> Subtract_47005/2
  Divide_b3bbc/1 -> Add_db1cd/1
  Subtract_4e4d5/1 -> Power_fbb4c/1
  State_psi_d_SG_D_22_1ab68/1 -> Add_db1cd/2
  Subtract_5b279/1 -> Subtract_5f8ae/1
  Constant_x_l_4e88b/1 -> Subtract_6b974/2
  Add_db1cd/1 -> Subtract_12a24/1
  Divide_58225/1 -> Subtract_12a24/2
  Constant_-1_be10d/1 -> Product_72ee2/1
  Product_f9d7f/1 -> Divide_eeebf/1
  State_psi_1d_SG_D_22_ea7d2/1 -> Product_72ee2/2
  Constant_x_dd_d9ba6/1 -> Subtract_6847d/1
  Constant_x_ddd_21800/1 -> Subtract_6847d/2
  Subtract_6b974/1 -> Product_8dcb9/1
  Subtract_12a24/1 -> Product_8dcb9/2
  Product_72ee2/1 -> Product_f9d7f/1
  Subtract_6847d/1 -> Product_f9d7f/2
  Constant_2.0_3cf32/1 -> Power_fbb4c/2
  Constant_x_dd_effc2/1 -> Subtract_8d9fd/1
  Constant_x_l_025b1/1 -> Subtract_8d9fd/2
  Constant_x_ddd_1b0fe/1 -> Subtract_1a20e/1
  Subtract_362e6/1 -> Product_95cd6/2
  Constant_x_dd_e67fe/1 -> Subtract_6c244/1
  Constant_x_dd_f4ac1/1 -> Subtract_362e6/1
  Constant_x_l_8603d/1 -> Subtract_1a20e/2
  Constant_x_l_4809b/1 -> Subtract_6c244/2
  State_psi_fd_SG_D_22_ee685/1 -> Product_9c35a/1
  State_psi_fd_SG_D_22_5b8ee/1 -> Subtract_5b279/2
  Constant_x_ddd_1deae/1 -> Subtract_362e6/2
  Subtract_f2eb4/1 -> Subtract_af608/1
  State_psi_1d_SG_D_22_be8ba/1 -> Subtract_f2eb4/1
  State_psi_fd_SG_D_22_f44ac/1 -> Subtract_f2eb4/2
  Product_8dcb9/1 -> Divide_05403/1
  Constant_x_ddd_45fea/1 -> Divide_05403/2
  Constant_x_l_d68d3/1 -> Subtract_4e4d5/2
  Subtract_8d9fd/1 -> Divide_eeebf/2
  Subtract_1a20e/1 -> Product_9c35a/2
  Divide_eeebf/1 -> Add_26b3d/1
  Constant_-1_84c87/1 -> Product_95cd6/1
  Divide_05403/1 -> Subtract_af608/2
  Constant_x_dd_31f3c/1 -> Subtract_4e4d5/1
  State_psi_d_SG_D_22_f7c75/1 -> Add_26b3d/2
  Product_9c35a/1 -> Divide_2963f/1
  Subtract_6c244/1 -> Divide_2963f/2
  Product_95cd6/1 -> Product_1b057/1
  Subtract_af608/1 -> Product_1b057/2
  Add_26b3d/1 -> Subtract_0684c/1
  Divide_2963f/1 -> Subtract_0684c/2
  Product_1b057/1 -> Divide_a0f43/1
  Power_fbb4c/1 -> Divide_a0f43/2
  Subtract_0684c/1 -> Divide_f671b/1
  Constant_x_ddd_e54ea/1 -> Divide_f671b/2
  Constant_x_d_d871a/1 -> Subtract_9e44c/1
  Constant_x_dd_b910b/1 -> Subtract_9e44c/2
  Divide_a0f43/1 -> Subtract_04006/1
  Divide_f671b/1 -> Subtract_04006/2
  Subtract_9e44c/1 -> Product_0db9f/1
  Subtract_04006/1 -> Product_0db9f/2
  Product_0db9f/1 -> Subtract_5f8ae/2
  Subtract_5f8ae/1 -> Divide_e4323/1
  Constant_T_dd_0394b/1 -> Divide_e4323/2
  Divide_e4323/1 -> Blockout_d_psi_fd_SG_D_22_1ac55/1

== system IEEE30_case/SG_D_22/d_psi_gq_SG_D_22_block ==
  note: d_psi_gq_SG_D_22 in IEEE30_case
      | $-\frac{\psi _{\mathrm{gq},\mathrm{SG},D,22}+\left(x_{q}-x_{\mathrm{qd}}\right)\,\left(\frac{\psi _{q,\mathrm{SG},D,22}+\frac{\psi _{\mathrm{gq},\mathrm{SG},D,22}\,\left(x_{l}-x_{\mathrm{qdd}}\right)}{x_{l}-x_{\mathrm{qd}}}+\frac{\psi _{\mathrm{kq},\mathrm{SG},D,22}\,\left(x_{\mathrm{qd}}-x_{\mathrm{qdd}}\right)}{x_{l}-x_{\mathrm{qd}}}}{x_{\mathrm{qdd}}}+\frac{\left(x_{\mathrm{qd}}-x_{\mathrm{qdd}}\right)\,\left(\psi _{\mathrm{gq},\mathrm{SG},D,22}+\psi _{\mathrm{kq},\mathrm{SG},D,22}+\frac{\left(x_{l}-x_{\mathrm{qd}}\right)\,\left(\psi _{q,\mathrm{SG},D,22}+\frac{\psi _{\mathrm{gq},\mathrm{SG},D,22}\,\left(x_{l}-x_{\mathrm{qdd}}\right)}{x_{l}-x_{\mathrm{qd}}}+\frac{\psi _{\mathrm{kq},\mathrm{SG},D,22}\,\left(x_{\mathrm{qd}}-x_{\mathrm{qdd}}\right)}{x_{l}-x_{\mathrm{qd}}}\right)}{x_{\mathrm{qdd}}}\right)}{{\left(x_{l}-x_{\mathrm{qd}}\right)}^2}\right)}{T_{\mathrm{qd}}}$
      | Automatically generated on 2025-11-01 18:36:07 .
  State_psi_gq_SG_D_22_18129 : Inport
  State_psi_gq_SG_D_22_c69e2 : Inport  Port=2
  State_psi_kq_SG_D_22_f3021 : Inport  Port=3
  State_psi_gq_SG_D_22_61da9 : Inport  Port=4
  State_psi_kq_SG_D_22_d52e6 : Inport  Port=5
  State_psi_q_SG_D_22_52758 : Inport  Port=6
  State_psi_gq_SG_D_22_1b6c4 : Inport  Port=7
  State_psi_kq_SG_D_22_c01c1 : Inport  Port=8
  State_psi_q_SG_D_22_91585 : Inport  Port=9
  Add_07d57 : Sum
  Add_2c990 : Sum
  Add_3abfb : Sum
  Add_6a1ab : Sum
  Add_87e36 : Sum
  Add_9ab8f : Sum
  Add_afbbb : Sum
  Add_b2a56 : Sum
  Add_bf692 : Sum
  Add_e5e4c : Sum
  Add_ecf83 : Sum
  Add_f2668 : Sum
  Constant_-1_1322b : Constant  Value=-1
  Constant_-1_17546 : Constant  Value=-1
  Constant_-1_29b0d : Constant  Value=-1
  Constant_-1_51805 : Constant  Value=-1
  Constant_-1_5262f : Constant  Value=-1
  Constant_-1_5de25 : Constant  Value=-1
  Constant_-1_86a5e : Constant  Value=-1
  Constant_-1_9b386 : Constant  Value=-1
  Constant_-1_ba96e : Constant  Value=-1
  Constant_-1_d3b63 : Constant  Value=-1
  Constant_2.0_730c0 : Constant  Value=2.0
  Constant_T_qd_bd741 : Constant  Value=T_qd
  Constant_x_l_031b1 : Constant  Value=x_l
  Constant_x_l_0e2d4 : Constant  Value=x_l
  Constant_x_l_31c01 : Constant  Value=x_l
  Constant_x_l_5bcd1 : Constant  Value=x_l
  Constant_x_l_60fcf : Constant  Value=x_l
  Constant_x_l_6842f : Constant  Value=x_l
  Constant_x_l_85f50 : Constant  Value=x_l
  Constant_x_l_e73c1 : Constant  Value=x_l
  Constant_x_q_1210a : Constant  Value=x_q
  Constant_x_qd_1e4a6 : Constant  Value=x_qd
  Constant_x_qd_2d894 : Constant  Value=x_qd
  Constant_x_qd_77cc5 : Constant  Value=x_qd
  Constant_x_qd_887b3 : Constant  Value=x_qd
  Constant_x_qd_8be9c : Constant  Value=x_qd
  Constant_x_qd_a1c48 : Constant  Value=x_qd
  Constant_x_qd_a3c16 : Constant  Value=x_qd
  Constant_x_qd_e76ab : Constant  Value=x_qd
  Constant_x_qd_fa2ec : Constant  Value=x_qd
  Constant_x_qd_fd7d8 : Constant  Value=x_qd
  Constant_x_qdd_06f8c : Constant  Value=x_qdd
  Constant_x_qdd_163b3 : Constant  Value=x_qdd
  Constant_x_qdd_71c9f : Constant  Value=x_qdd
  Constant_x_qdd_9365f : Constant  Value=x_qdd
  Constant_x_qdd_9bf1c : Constant  Value=x_qdd
  Constant_x_qdd_a5256 : Constant  Value=x_qdd
  Constant_x_qdd_ea269 : Constant  Value=x_qdd
  Divide_06e20 : Product  Inputs=*/
  Divide_62c8d : Product  Inputs=*/
  Divide_63053 : Product  Inputs=*/
  Divide_66c94 : Product  Inputs=*/
  Divide_8576e : Product  Inputs=*/
  Divide_c0123 : Product  Inputs=*/
  Divide_c85fd : Product  Inputs=*/
  Divide_e4bc8 : Product  Inputs=*/
  Power_ac163 : Math  Operator=pow
  Product_097c3 : Product
  Product_29b15 : Product
  Product_35b90 : Product
  Product_5303f : Product
  Product_5bbbe : Product
  Product_7d146 : Product
  Product_7f589 : Product
  Product_8a4af : Product
  Product_97702 : Product
  Product_cce46 : Product
  Product_ce041 : Product
  Product_d0653 : Product
  Product_dcb71 : Product
  Product_ddb40 : Product
  Product_f0eb2 : Product
  Product_f7dcf : Product
  Product_fa634 : Product
  Subtract_0e545 : Sum  Inputs=+-
  Subtract_1f065 : Sum  Inputs=+-
  Subtract_47138 : Sum  Inputs=+-
  Subtract_716d0 : Sum  Inputs=+-
  Subtract_9dab1 : Sum  Inputs=+-
  Subtract_cb47e : Sum  Inputs=+-
  Subtract_ce2d9 : Sum  Inputs=+-
  Subtract_fa774 : Sum  Inputs=+-
  Blockout_d_psi_gq_SG_D_22_8bac2 : Outport
  wires:
  Constant_x_qdd_ea269/1 -> Add_07d57/2
  State_psi_gq_SG_D_22_c69e2/1 -> Add_87e36/1
  State_psi_kq_SG_D_22_c01c1/1 -> Product_ce041/1
  Constant_x_qdd_a5256/1 -> Subtract_9dab1/2
  Constant_-1_51805/1 -> Product_d0653/1
  Product_d0653/1 -> Add_07d57/1
  Subtract_fa774/1 -> Product_97702/2
  Product_ce041/1 -> Divide_62c8d/1
  Constant_x_l_031b1/1 -> Product_d0653/2
  Product_5303f/1 -> Add_6a1ab/1
  Constant_-1_86a5e/1 -> Product_5303f/1
  Subtract_cb47e/1 -> Product_35b90/2
  Constant_x_qd_887b3/1 -> Subtract_cb47e/1
  Add_ecf83/1 -> Divide_62c8d/2
  Product_7d146/1 -> Divide_06e20/1
  Constant_x_l_5bcd1/1 -> Product_5303f/2
  Constant_x_qdd_9365f/1 -> Subtract_cb47e/2
  Product_cce46/1 -> Add_b2a56/1
  Constant_-1_5de25/1 -> Product_cce46/1
  Constant_x_l_e73c1/1 -> Product_cce46/2
  Constant_x_l_0e2d4/1 -> Product_f0eb2/2
  Product_8a4af/1 -> Divide_c85fd/1
  State_psi_gq_SG_D_22_61da9/1 -> Product_8a4af/1
  State_psi_kq_SG_D_22_f3021/1 -> Add_87e36/2
  Add_07d57/1 -> Product_8a4af/2
  Constant_x_qd_8be9c/1 -> Add_6a1ab/2
  Product_35b90/1 -> Divide_e4bc8/1
  State_psi_kq_SG_D_22_d52e6/1 -> Product_35b90/1
  Constant_x_qd_2d894/1 -> Add_b2a56/2
  Constant_x_l_60fcf/1 -> Product_097c3/2
  Add_6a1ab/1 -> Divide_c85fd/2
  Add_b2a56/1 -> Divide_e4bc8/2
  Constant_-1_29b0d/1 -> Product_5bbbe/1
  Add_f2668/1 -> Divide_8576e/2
  Constant_x_qd_a3c16/1 -> Add_ecf83/2
  Constant_x_l_31c01/1 -> Product_5bbbe/2
  Divide_c85fd/1 -> Subtract_716d0/1
  Divide_e4bc8/1 -> Subtract_716d0/2
  State_psi_q_SG_D_22_52758/1 -> Add_2c990/2
  Constant_-1_5262f/1 -> Product_29b15/1
  Constant_x_l_85f50/1 -> Product_29b15/2
  Constant_-1_17546/1 -> Product_097c3/1
  Product_5bbbe/1 -> Add_3abfb/1
  Product_f0eb2/1 -> Add_f2668/1
  Constant_x_qd_1e4a6/1 -> Add_3abfb/2
  Constant_x_qdd_06f8c/1 -> Subtract_0e545/2
  Subtract_716d0/1 -> Add_2c990/1
  Product_29b15/1 -> Add_9ab8f/1
  Constant_x_qdd_71c9f/1 -> Add_9ab8f/2
  Constant_-1_ba96e/1 -> Product_7f589/1
  Constant_-1_d3b63/1 -> Product_f0eb2/1
  Constant_x_qd_e76ab/1 -> Subtract_9dab1/1
  Product_097c3/1 -> Add_ecf83/1
  Add_3abfb/1 -> Product_7d146/1
  Add_2c990/1 -> Product_7d146/2
  Constant_x_qdd_163b3/1 -> Divide_06e20/2
  State_psi_gq_SG_D_22_1b6c4/1 -> Product_fa634/1
  Add_9ab8f/1 -> Product_fa634/2
  Constant_x_qd_77cc5/1 -> Add_f2668/2
  Subtract_9dab1/1 -> Product_ce041/2
  Subtract_0e545/1 -> Product_7f589/2
  Constant_x_qd_a1c48/1 -> Subtract_0e545/1
  Constant_-1_9b386/1 -> Product_ddb40/1
  Constant_x_l_6842f/1 -> Product_ddb40/2
  Product_fa634/1 -> Divide_8576e/1
  Add_87e36/1 -> Subtract_fa774/1
  Divide_06e20/1 -> Subtract_fa774/2
  Product_ddb40/1 -> Add_e5e4c/1
  Constant_x_qd_fa2ec/1 -> Add_e5e4c/2
  Divide_8576e/1 -> Subtract_47138/1
  Constant_T_qd_bd741/1 -> Divide_66c94/2
  Divide_62c8d/1 -> Subtract_47138/2
  Product_7f589/1 -> Product_97702/1
  Add_e5e4c/1 -> Power_ac163/1
  Constant_2.0_730c0/1 -> Power_ac163/2
  Subtract_47138/1 -> Add_bf692/1
  State_psi_q_SG_D_22_91585/1 -> Add_bf692/2
  Product_97702/1 -> Divide_63053/1
  Power_ac163/1 -> Divide_63053/2
  Add_bf692/1 -> Divide_c0123/1
  Constant_x_qdd_9bf1c/1 -> Divide_c0123/2
  Constant_x_q_1210a/1 -> Subtract_ce2d9/1
  Constant_x_qd_fd7d8/1 -> Subtract_ce2d9/2
  Divide_63053/1 -> Subtract_1f065/1
  Divide_c0123/1 -> Subtract_1f065/2
  Constant_-1_1322b/1 -> Product_f7dcf/1
  State_psi_gq_SG_D_22_18129/1 -> Product_f7dcf/2
  Subtract_ce2d9/1 -> Product_dcb71/1
  Subtract_1f065/1 -> Product_dcb71/2
  Product_f7dcf/1 -> Add_afbbb/1
  Product_dcb71/1 -> Add_afbbb/2
  Add_afbbb/1 -> Divide_66c94/1
  Divide_66c94/1 -> Blockout_d_psi_gq_SG_D_22_8bac2/1

== system IEEE30_case/SG_D_22/d_psi_kq_SG_D_22_block ==
  note: d_psi_kq_SG_D_22 in IEEE30_case
      | $-\frac{\psi _{\mathrm{gq},\mathrm{SG},D,22}+\psi _{\mathrm{kq},\mathrm{SG},D,22}+\frac{\left(x_{l}-x_{\mathrm{qd}}\right)\,\left(\psi _{q,\mathrm{SG},D,22}+\frac{\psi _{\mathrm{gq},\mathrm{SG},D,22}\,\left(x_{l}-x_{\mathrm{qdd}}\right)}{x_{l}-x_{\mathrm{qd}}}+\frac{\psi _{\mathrm{kq},\mathrm{SG},D,22}\,\left(x_{\mathrm{qd}}-x_{\mathrm{qdd}}\right)}{x_{l}-x_{\mathrm{qd}}}\right)}{x_{\mathrm{qdd}}}}{T_{\mathrm{qdd}}}$
      | Automatically generated on 2025-11-01 18:36:10 .
  State_psi_gq_SG_D_22_5f63f : Inport
  State_psi_kq_SG_D_22_eb2c5 : Inport  Port=2
  State_psi_gq_SG_D_22_c1d1e : Inport  Port=3
  State_psi_kq_SG_D_22_49ea5 : Inport  Port=4
  State_psi_q_SG_D_22_89f21 : Inport  Port=5
  Add_0036d : Sum
  Add_1524c : Sum
  Add_34349 : Sum
  Add_6f465 : Sum
  Add_9cd98 : Sum
  Add_cc277 : Sum
  Constant_-1_01350 : Constant  Value=-1
  Constant_-1_1a4c9 : Constant  Value=-1
  Constant_-1_64fa4 : Constant  Value=-1
  Constant_-1_c1ae2 : Constant  Value=-1
  Constant_-1_eed7c : Constant  Value=-1
  Constant_T_qdd_0d458 : Constant  Value=T_qdd
  Constant_x_l_39cec : Constant  Value=x_l
  Constant_x_l_6c12c : Constant  Value=x_l
  Constant_x_l_b70cb : Constant  Value=x_l
  Constant_x_l_ecc30 : Constant  Value=x_l
  Constant_x_qd_05283 : Constant  Value=x_qd
  Constant_x_qd_08905 : Constant  Value=x_qd
  Constant_x_qd_7aa12 : Constant  Value=x_qd
  Constant_x_qd_a45eb : Constant  Value=x_qd
  Constant_x_qdd_2b27a : Constant  Value=x_qdd
  Constant_x_qdd_3bf1e : Constant  Value=x_qdd
  Constant_x_qdd_da78e : Constant  Value=x_qdd
  Divide_9e01a : Product  Inputs=*/
  Divide_b7239 : Product  Inputs=*/
  Divide_be0c6 : Product  Inputs=*/
  Divide_ef790 : Product  Inputs=*/
  Product_1e44e : Product
  Product_60e22 : Product
  Product_72460 : Product
  Product_7b858 : Product
  Product_ae435 : Product
  Product_b6c5f : Product
  Product_cc7f6 : Product
  Product_ec9b0 : Product
  Subtract_36676 : Sum  Inputs=+-
  Subtract_918e8 : Sum  Inputs=+-
  Subtract_e7932 : Sum  Inputs=+-
  Blockout_d_psi_kq_SG_D_22_a4b99 : Outport
  wires:
  Product_b6c5f/1 -> Add_cc277/1
  Constant_-1_c1ae2/1 -> Product_b6c5f/1
  Constant_-1_01350/1 -> Product_7b858/1
  State_psi_q_SG_D_22_89f21/1 -> Add_34349/2
  Constant_-1_64fa4/1 -> Product_60e22/1
  Product_ae435/1 -> Add_6f465/1
  Constant_-1_1a4c9/1 -> Product_ae435/1
  Constant_x_l_ecc30/1 -> Product_7b858/2
  Product_ec9b0/1 -> Divide_be0c6/1
  Subtract_918e8/1 -> Product_1e44e/2
  Constant_x_qd_05283/1 -> Subtract_918e8/1
  Constant_x_l_b70cb/1 -> Product_b6c5f/2
  Constant_x_qdd_3bf1e/1 -> Add_9cd98/2
  Product_7b858/1 -> Add_9cd98/1
  Constant_x_qdd_2b27a/1 -> Subtract_918e8/2
  Constant_x_l_39cec/1 -> Product_ae435/2
  State_psi_gq_SG_D_22_c1d1e/1 -> Product_72460/1
  Add_9cd98/1 -> Product_72460/2
  Divide_ef790/1 -> Subtract_36676/1
  Constant_x_qd_08905/1 -> Add_cc277/2
  Constant_-1_eed7c/1 -> Product_cc7f6/1
  Product_1e44e/1 -> Divide_b7239/1
  State_psi_kq_SG_D_22_49ea5/1 -> Product_1e44e/1
  Constant_x_qd_7aa12/1 -> Add_6f465/2
  Product_72460/1 -> Divide_ef790/1
  Add_0036d/1 -> Divide_9e01a/1
  Add_cc277/1 -> Divide_ef790/2
  State_psi_kq_SG_D_22_eb2c5/1 -> Subtract_e7932/2
  Add_6f465/1 -> Divide_b7239/2
  Divide_9e01a/1 -> Blockout_d_psi_kq_SG_D_22_a4b99/1
  Constant_x_l_6c12c/1 -> Product_60e22/2
  Product_cc7f6/1 -> Subtract_e7932/1
  Divide_b7239/1 -> Subtract_36676/2
  Product_60e22/1 -> Add_1524c/1
  Constant_x_qd_a45eb/1 -> Add_1524c/2
  Subtract_36676/1 -> Add_34349/1
  State_psi_gq_SG_D_22_5f63f/1 -> Product_cc7f6/2
  Add_1524c/1 -> Product_ec9b0/1
  Add_34349/1 -> Product_ec9b0/2
  Constant_x_qdd_da78e/1 -> Divide_be0c6/2
  Subtract_e7932/1 -> Add_0036d/1
  Divide_be0c6/1 -> Add_0036d/2
  Constant_T_qdd_0d458/1 -> Divide_9e01a/2

== system IEEE30_case/SG_D_22/d_psi_q_SG_D_22_block ==
  note: d_psi_q_SG_D_22 in IEEE30_case
      | $2\,\pi \,f_{0}\,\left(v_{d,\mathrm{SG},D,22}\,\cos\left(\theta _{\mathrm{SG},D,22}\right)+v_{q,\mathrm{SG},D,22}\,\sin\left(\theta _{\mathrm{SG},D,22}\right)-\frac{R_{a}\,\left(\psi _{q,\mathrm{SG},D,22}+\frac{\psi _{\mathrm{gq},\mathrm{SG},D,22}\,\left(x_{l}-x_{\mathrm{qdd}}\right)}{x_{l}-x_{\mathrm{qd}}}+\frac{\psi _{\mathrm{kq},\mathrm{SG},D,22}\,\left(x_{\mathrm{qd}}-x_{\mathrm{qdd}}\right)}{x_{l}-x_{\mathrm{qd}}}\right)}{x_{\mathrm{qdd}}}-\frac{\psi _{d,\mathrm{SG},D,22}\,w_{\mathrm{SG},D,22}}{2\,f_{0}\,\pi }\right)$
      | Automatically generated on 2025-11-01 18:35:53 .
  State_psi_gq_SG_D_22_8eb30 : Inport
  State_psi_kq_SG_D_22_098fe : Inport  Port=2
  State_psi_q_SG_D_22_dc44e : Inport  Port=3
  Input_v_d_SG_D_22_2b34c : Inport  Port=4
  State_theta_SG_D_22_55bda : Inport  Port=5
  Input_v_q_SG_D_22_03d27 : Inport  Port=6
  State_theta_SG_D_22_3fd59 : Inport  Port=7
  State_psi_d_SG_D_22_a1733 : Inport  Port=8
  State_w_SG_D_22_27ecd : Inport  Port=9
  Add_41198 : Sum
  Add_67836 : Sum
  Add_68403 : Sum
  Add_76ce4 : Sum
  Add_bd123 : Sum
  Constant_-1_919ff : Constant  Value=-1
  Constant_-1_c9b65 : Constant  Value=-1
  Constant_-1_d6dc4 : Constant  Value=-1
  Constant_-2.0_801fc : Constant  Value=-2.0
  Constant_2.0_e7afa : Constant  Value=2.0
  Constant_R_a_6b14d : Constant  Value=R_a
  Constant_f0_03cc4 : Constant  Value=f0
  Constant_f0_e2cd3 : Constant  Value=f0
  Constant_pi_4f685 : Constant  Value=pi
  Constant_pi_9c1d5 : Constant  Value=pi
  Constant_x_l_39a61 : Constant  Value=x_l
  Constant_x_l_6c18d : Constant  Value=x_l
  Constant_x_l_7a427 : Constant  Value=x_l
  Constant_x_qd_03fd2 : Constant  Value=x_qd
  Constant_x_qd_0d235 : Constant  Value=x_qd
  Constant_x_qd_d9f67 : Constant  Value=x_qd
  Constant_x_qdd_49a8e : Constant  Value=x_qdd
  Constant_x_qdd_5dcad : Constant  Value=x_qdd
  Constant_x_qdd_ade8b : Constant  Value=x_qdd
  Divide_3f603 : Product  Inputs=*/
  Divide_548c1 : Product  Inputs=*/
  Divide_8299a : Product  Inputs=*/
  Divide_e5f8c : Product  Inputs=*/
  MathFunc_cos_79477 : Trigonometry  Operator=cos
  MathFunc_sin_97ad2 : Trigonometry
  Product_0579a : Product
  Product_0705f : Product
  Product_0d01b : Product
  Product_1fe4b : Product
  Product_1ff36 : Product
  Product_21c70 : Product
  Product_2c9d2 : Product
  Product_636cf : Product
  Product_8377d : Product
  Product_8654a : Product
  Product_bcacb : Product
  Product_be755 : Product
  Product_d0fc6 : Product
  Product_e1676 : Product
  Subtract_58713 : Sum  Inputs=+-
  Subtract_5d666 : Sum  Inputs=+-
  Subtract_ccf8c : Sum  Inputs=+-
  Subtract_ec504 : Sum  Inputs=+-
  Blockout_d_psi_q_SG_D_22_d620a : Outport
  wires:
  Constant_-1_919ff/1 -> Product_8654a/1
  Constant_x_l_7a427/1 -> Product_8654a/2
  Constant_f0_e2cd3/1 -> Product_d0fc6/2
  Constant_x_l_6c18d/1 -> Product_be755/2
  Product_8654a/1 -> Add_76ce4/1
  Subtract_ec504/1 -> Subtract_ccf8c/1
  Constant_x_qdd_5dcad/1 -> Add_76ce4/2
  Divide_e5f8c/1 -> Subtract_ec504/1
  Add_41198/1 -> Product_0705f/2
  Constant_-1_d6dc4/1 -> Product_be755/1
  Subtract_58713/1 -> Add_41198/1
  Constant_x_qd_0d235/1 -> Subtract_5d666/1
  Constant_-2.0_801fc/1 -> Product_bcacb/1
  Constant_x_qdd_49a8e/1 -> Subtract_5d666/2
  Product_e1676/1 -> Blockout_d_psi_q_SG_D_22_d620a/1
  Constant_f0_03cc4/1 -> Product_2c9d2/2
  Constant_-1_c9b65/1 -> Product_21c70/1
  Constant_x_l_39a61/1 -> Product_21c70/2
  State_psi_gq_SG_D_22_8eb30/1 -> Product_1fe4b/1
  Add_76ce4/1 -> Product_1fe4b/2
  Product_be755/1 -> Add_67836/1
  Constant_x_qd_d9f67/1 -> Add_67836/2
  State_psi_kq_SG_D_22_098fe/1 -> Product_0d01b/1
  Subtract_5d666/1 -> Product_0d01b/2
  Product_d0fc6/1 -> Product_e1676/1
  Constant_pi_9c1d5/1 -> Product_1ff36/2
  Product_0705f/1 -> Divide_e5f8c/1
  Product_21c70/1 -> Add_68403/1
  Product_2c9d2/1 -> Divide_3f603/2
  Constant_x_qd_03fd2/1 -> Add_68403/2
  Subtract_ccf8c/1 -> Add_bd123/1
  Product_1fe4b/1 -> Divide_548c1/1
  Add_67836/1 -> Divide_548c1/2
  Product_0d01b/1 -> Divide_8299a/1
  Add_68403/1 -> Divide_8299a/2
  Divide_548c1/1 -> Subtract_58713/1
  Divide_8299a/1 -> Subtract_58713/2
  State_psi_q_SG_D_22_dc44e/1 -> Add_41198/2
  Constant_R_a_6b14d/1 -> Product_0705f/1
  MathFunc_cos_79477/1 -> Product_8377d/2
  State_theta_SG_D_22_55bda/1 -> MathFunc_cos_79477/1
  Constant_x_qdd_ade8b/1 -> Divide_e5f8c/2
  Product_8377d/1 -> Subtract_ec504/2
  Input_v_d_SG_D_22_2b34c/1 -> Product_8377d/1
  State_theta_SG_D_22_3fd59/1 -> MathFunc_sin_97ad2/1
  Constant_2.0_e7afa/1 -> Product_1ff36/1
  Input_v_q_SG_D_22_03d27/1 -> Product_636cf/1
  MathFunc_sin_97ad2/1 -> Product_636cf/2
  Product_bcacb/1 -> Product_d0fc6/1
  Product_0579a/1 -> Divide_3f603/1
  State_psi_d_SG_D_22_a1733/1 -> Product_0579a/1
  State_w_SG_D_22_27ecd/1 -> Product_0579a/2
  Product_1ff36/1 -> Product_2c9d2/1
  Constant_pi_4f685/1 -> Product_bcacb/2
  Product_636cf/1 -> Subtract_ccf8c/2
  Divide_3f603/1 -> Add_bd123/2
  Add_bd123/1 -> Product_e1676/2

== system IEEE30_case/SG_D_22/d_theta_SG_D_22_block ==
  note: d_theta_SG_D_22 in IEEE30_case
      | $w_{\mathrm{SG},D,22}-2\,\pi \,f_{0}$
      | Automatically generated on 2025-11-01 18:36:17 .
  State_w_SG_D_22_7f5ca : Inport
  Add_24169 : Sum
  Constant_-2.0_0f3c7 : Constant  Value=-2.0
  Constant_f0_4ea11 : Constant  Value=f0
  Constant_pi_87fb7 : Constant  Value=pi
  Product_a0416 : Product
  Product_e17e8 : Product
  Blockout_d_theta_SG_D_22_65d2b : Outport
  wires:
  Constant_-2.0_0f3c7/1 -> Product_a0416/1
  Constant_pi_87fb7/1 -> Product_a0416/2
  Product_a0416/1 -> Product_e17e8/1
  Constant_f0_4ea11/1 -> Product_e17e8/2
  Add_24169/1 -> Blockout_d_theta_SG_D_22_65d2b/1
  Product_e17e8/1 -> Add_24169/1
  State_w_SG_D_22_7f5ca/1 -> Add_24169/2
